simulink model "Quadruped"  (R2020a)
settings: Solver=VariableStepAuto  StartTime=0.0  StopTime=10.0  RelTol=1e-3  EnableMultiTasking=on
PreLoadFcn:
  | Parameters;
values from neighbouring files (symbols this model uses):
  buffer = 8000    [Parameters.m]
  gait_time = 1    [Parameters.m]
  l1 = 0.2    [Parameters.m]
  l2 = 0.4    [Parameters.m]
  l3 = l3_orig-r    (= 0.38)    [Parameters.m]
  robot_b = 0.1    [Parameters.m]
  robot_l = 1    [Parameters.m]
  robot_w = 0.4    [Parameters.m]
  step_height = 0.1    [Parameters.m]
  step_time = gait_time/2    (= 0.5)    [Parameters.m]
  target1 = 0    [Parameters.m]
  target2 = 30    [Parameters.m]
  target2r = -30    [Parameters.m]
  target3 = -120    [Parameters.m]
  target3r = 120    [Parameters.m]
  Xc_i = 0    [Parameters.m]
undefined symbols (not defined in the file or in its folder): X, Y, Z
libraries: sm_lib x76, nesl_utility x46, simulink x26
(part 1 of 4)
settings Model: Creator=user  LastModifiedBy=ashut
settings DataIOCC: LimitDataPoints=on  MaxDataPoints=10000
settings OptimizationCC: LifeSpan=inf
settings DebuggingCC: AllowSymbolicDim=off  SFUnexpectedBacktrackingDiag=warning  SFNoUnconditionalDefaultTransitionDiag=warning  SFExecutionAtInitializationDiag=none  ArithmeticOperatorsInVariantConditions=warning
settings SFSimCC: SimUseLocalCustomCode=off  CustomCodeUndefinedFunction=UseInterfaceOnly
settings RTWCC: RTWUseLocalCustomCode=off
settings CodeAppCC: StateflowObjectComments=on
settings GRTTargetCC: TargetLangStandard=C89/C90 (ANSI)
settings ConfigComp: CovMetricSettings=dw  CovHtmlReporting=on  CovSaveCumulativeToWorkspaceVar=on  CovSaveSingleToWorkspaceVar=on  CovExternalEMLEnable=off  CovSFcnEnable=off
settings SimscapeCC: SimscapeLogType=all  SimscapeLogSimulationStatistics=on  SimscapeLogDataHistory=10000
settings ExplorerConfigSet: InternalSimMechanicsExplorerSettings="<ExplorerConfiguration><canonicalview>default</canonicalview><AnimationSetting><BasePlaybackSpeed>1.0</BasePlaybackSpeed><PlaybackSpeedFactor>1.0</PlaybackSpeedFactor></AnimationSetting><TilePanel><TileInfo><Tiles Columns=\"1\" Count=\"1\" Rows=\"1\"><Column Weight=\"1\"/><Row Weight=\"1\"/><Tile Height=\"1\" Width=\"1\" X=\"0\" Y=\"0\"/></Tiles></TileInfo><SceneInfo><SceneViewer><BGColor><R>0.60000002384185791</R><G>0.60000002384185791</G><B>0.60000002384185791</B></BGColor><Camera><DoPerspective>off</DoPerspective><Position><X>29.2456293007888846</X><Y>-28.7629640651694523</Y><Z>29.0332714283084741</Z></Position><Center><X>0.231674806078519896</X><Y>0.250990429540917881</Y><Z>0.0193169335981059412</Z></Center><Up><X>-0.408248290463863073</X><Y>0.408248290463863073</Y><Z>0.816496580927726145</Z></Up><ViewLimDist>1</ViewLimDist><YLim>1.3149570353676332</YLim><XLim>2.00111393750615596</XLim></Camera></SceneViewer></SceneInfo></TilePanel><MechEditorPanel><Cameras/><GfxPanelCameraMap/><VideoCreator><PlaybackSpeedRatio>1.0</PlaybackSpeedRatio><FrameRate>30</FrameRate><VideoFormat>Motion JPEG AVI</VideoFormat><FrameSize>auto</FrameSize></VideoCreator></MechEditorPanel></ExplorerConfiguration>"

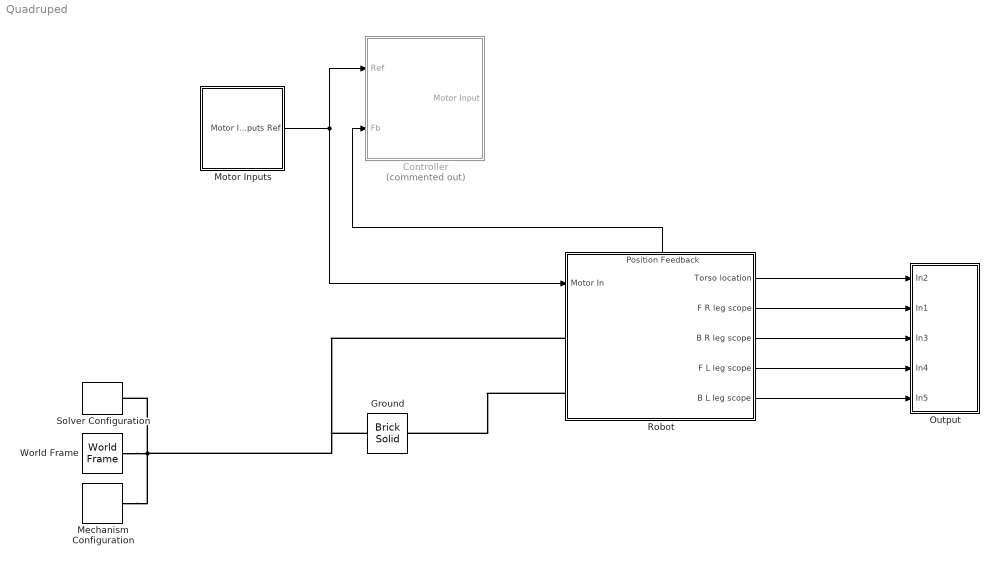
== system Quadruped ==
  Controller : Subsystem  Commented=on
  Ground : sm_lib/Body Elements/Brick Solid  GraphicAmbientColor=[0.15 0.15 0.15 1.0]  BasedOnType=Density  BrickDimensions=[100 5 0.1]  BrickDimensionUnits=m  CenterOfMass=[0 0 0]  CenterOfMassUnits=m  GraphicDiffuseColor=[0.5 0.5 0.5]  Density=1000  DensityUnits=kg/m^3  DoExposeReferenceFrame=on  GraphicEmissiveColor=[0.0 0.0 0.0 1.0]  ExportEntireGeometry=on  SerializedFrames=<Frames/>  MarkerShape=Sphere  MarkerSize=10  GraphicType=FromGeometry  InertiaType=CalculateFromGeometry  Mass=1  MassUnits=kg  MomentsOfInertia=[1 1 1]  MomentsOfInertiaUnits=kg*m^2  GraphicOpacity=1.0  ProductsOfInertia=[0 0 0]  ProductsOfInertiaUnits=kg*m^2  GraphicShininess=75  GraphicSpecularColor=[0.5 0.5 0.5 1.0]  GraphicVisPropType=SimpleVisualProperties
  Mechanism Configuration : sm_lib/Utilities/Mechanism Configuration  UniformGravity=Constant  GravityVector=[0 0 -9.8066]  GravityUnits=m/s^2  LinearizationDelta=0.001
  Motor Inputs : Subsystem
  Output : Subsystem
  Robot : Subsystem
      settings: PortSchema="{\"entries\":[{\"content\":{\"sides\":[{\"content\":{\"connectorIds\":[\"In1\",\"LConn1\",\"LConn2\"]},\"type\":\"ConnectorPlacement.EquallySpacedRectSide\",\"uuid\":\"4635b272-c60d-4014-ab6c-106026f55e73\"},{\"content\":{\"connectorIds\":[\"Out1\",\"Out2\",\"Out3\",\"Out4\",\"Out5\"],\"side\":\"RIGHT\"},\"type\":\"ConnectorPlacement.EquallySpacedRectSide\",\"uuid\":\"ef84d230-707b-4f1f-8f8a-5325fbe6d1ad\"},{\"content\":{\"connectorIds\":[\"Out6\"],\"side\":\"TOP\"},\"type\":\"ConnectorPlacement.EquallySpacedRectSide\",\"uuid\":\"c3e351c9-2d6a-4656-b5fa-3d004952b50f\"}]},\"type\":\"ConnectorPlacement.EquallySpacedConnector\",\"uuid\":\"b3bf907b-4dd7-42ee-b13b-00e04b6696fd\"}],\"packageUris\":[\"http://schema.mathworks.com/mf0/Connector/19700101\"],\"version\":\"1.0\"}"
  Solver Configuration : nesl_utility/Solver Configuration  PhysicalDomain=network_engine_domain  SubClassName=solver  LeftPortType=input  RightPortType=generic  Tones=[]  Harmonics=[]  SimulateNoise=off  Profile=off  UseLocalSampling=off  EnableSwitchedLinearOptims=on  FrequencyDomain=off  UseCCode=off  RelTol=0.001  AbsTol=1e-06  MinStep=1e-09  ToWorkspace=off  RevertToSquareIcSolve=off  NumHomotopyIterations=100  PhasorMode=off  PhasorModeNumHarmonics=1  DoDC=off  ResidualTolerance=1e-09  UseLocalSolver=off  LocalSolverChoice=NE_BACKWARD_EULER_ADVANCER  LocalSolverSampleTime=0.001  DoFixedCost=off  MaxNonlinIter=3  MaxModeIter=2  LinearAlgebra=Sparse  EquationFormulation=NE_TIME_EF  DelaysMemoryBudget=1024  AutomaticFiltering=on  FilteringTimeConstant=0.001  PartitionStorageMethod=AS_NEEDED  PartitionMemoryBudget=1024  PartitionMethod=FAST
  World Frame : sm_lib/Frames and Transforms/World Frame
  wires:
  Robot/2(F R leg scope) -> Output/2(In1)
  Robot/1(Torso location) -> Output/1(In2)
  Robot/3(B R leg scope) -> Output/3(In3)
  Robot/4(F L leg scope) -> Output/4(In4)
  Robot/5(B L leg scope) -> Output/5(In5)
  Motor Inputs/1(Motor Inputs Ref) -> Robot/1(Motor In), Controller/1(Ref)
  Robot/6(Position Feedback) -> Controller/2(Fb)
  connections:
  World Frame/RConn1 -- Ground/RConn1 -- Robot/LConn1 -- Solver Configuration/RConn1 -- Mechanism Configuration/RConn1
  Robot/LConn2 -- Ground/LConn1

== system Quadruped/Controller ==
  Ref : Inport
  Fb : Inport  Port=2
  Simple PID for each motor : Subsystem
  Motor Input : Outport
  wires:
  Ref/1 -> Simple PID for each motor/1(Ref)
  Fb/1 -> Simple PID for each motor/2(Fb)
  Simple PID for each motor/1(Motor Input) -> Motor Input/1

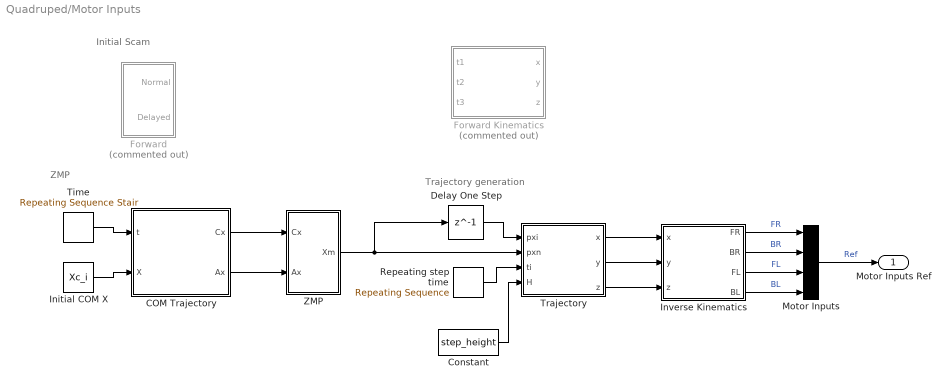
== system Quadruped/Motor Inputs ==
  note: Trajectory generation
  note: ZMP
  note: Initial Scam
  COM Trajectory : MATLAB Function  TreatAsAtomicUnit=on
  Constant : Constant  Value=step_height
  Delay One Step : Delay  DelayLength=1
  Forward : Subsystem  Commented=on
  Forward Kinematics : MATLAB Function  Commented=on  TreatAsAtomicUnit=on
  Initial COM X : Constant  Value=Xc_i
  Inverse Kinematics : Subsystem
  Motor Inputs : BusCreator  Inputs=4
  Repeating step time : simulink/Sources/Repeating Sequence  rep_seq_t=[0 step_time]  rep_seq_y=[0 step_time]
  Time : simulink/Sources/Repeating Sequence Stair  OutValues=[0:gait_time:10].'  tsamp=gait_time  OutMin=[]  OutMax=[]  OutDataTypeStr=double  OutputDataTypeScalingMode=double  OutDataType=fixdt(0,8)  ConRadixGroup=Best Precision: Vector-wise  OutScaling=2^-12
  Trajectory : MATLAB Function  TreatAsAtomicUnit=on
  ZMP : MATLAB Function  TreatAsAtomicUnit=on
  Motor Inputs Ref : Outport
  wires:
  COM Trajectory/1(Cx) -> ZMP/1(Cx)
  COM Trajectory/2(Ax) -> ZMP/2(Ax)
  Trajectory/3(z) -> Inverse Kinematics/3(z)
  Trajectory/2(y) -> Inverse Kinematics/2(y)
  Trajectory/1(x) -> Inverse Kinematics/1(x)
  Constant/1 -> Trajectory/4(H)
  Inverse Kinematics/1(FR) -> Motor Inputs/1  "FR"
  Inverse Kinematics/2(BR) -> Motor Inputs/2  "BR"
  Inverse Kinematics/3(FL) -> Motor Inputs/3  "FL"
  Inverse Kinematics/4(BL) -> Motor Inputs/4  "BL"
  Motor Inputs/1 -> Motor Inputs Ref/1  "Ref"
  Initial COM X/1 -> COM Trajectory/2(X)
  Time/1 -> COM Trajectory/1(t)
  Repeating step time/1 -> Trajectory/3(ti)
  ZMP/1(Xm) -> Delay One Step/1, Trajectory/2(pxn)
  Delay One Step/1 -> Trajectory/1(pxi)

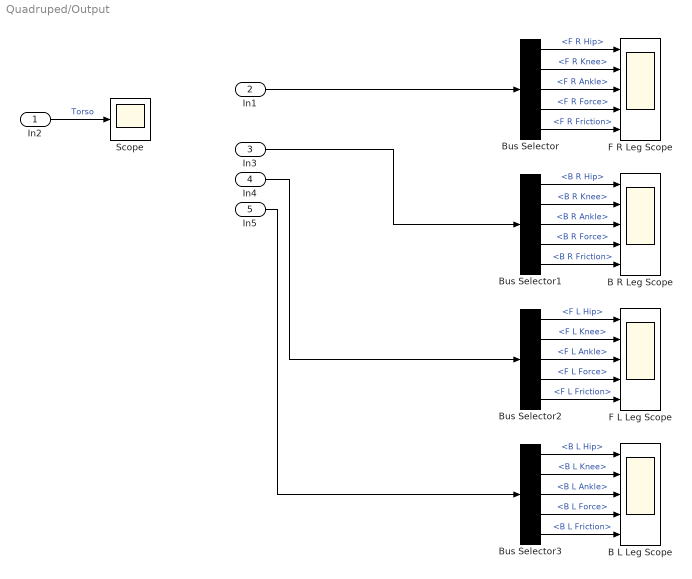
== system Quadruped/Output ==
  In2 : Inport
  In1 : Inport  Port=2
  In3 : Inport  Port=3
  In4 : Inport  Port=4
  In5 : Inport  Port=5
  B L Leg Scope : Scope  NumInputPorts=5
  B R Leg Scope : Scope  NumInputPorts=5
  Bus Selector : BusSelector  OutputSignals=Torques & Force.F R Hip,Torques & Force.F R Knee,Torques & Force.F R Ankle,Torques & Force.F R Force,Torques & Force.F R Friction
  Bus Selector1 : BusSelector  OutputSignals=Torques & Force.B R Hip,Torques & Force.B R Knee,Torques & Force.B R Ankle,Torques & Force.B R Force,Torques & Force.B R Friction
  Bus Selector2 : BusSelector  OutputSignals=Torques & Force.F L Hip,Torques & Force.F L Knee,Torques & Force.F L Ankle,Torques & Force.F L Force,Torques & Force.F L Friction
  Bus Selector3 : BusSelector  OutputSignals=Torques & Force.B L Hip,Torques & Force.B L Knee,Torques & Force.B L Ankle,Torques & Force.B L Force,Torques & Force.B L Friction
  F L Leg Scope : Scope  NumInputPorts=5
  F R Leg Scope : Scope  NumInputPorts=5
  Scope : Scope
  wires:
  Bus Selector2/2 -> F L Leg Scope/2  "<F L Knee>"
  Bus Selector3/3 -> B L Leg Scope/3  "<B L Ankle>"
  Bus Selector1/3 -> B R Leg Scope/3  "<B R Ankle>"
  Bus Selector3/2 -> B L Leg Scope/2  "<B L Knee>"
  Bus Selector1/1 -> B R Leg Scope/1  "<B R Hip>"
  In1/1 -> Bus Selector/1
  Bus Selector2/4 -> F L Leg Scope/4  "<F L Force>"
  Bus Selector1/2 -> B R Leg Scope/2  "<B R Knee>"
  Bus Selector/1 -> F R Leg Scope/1  "<F R Hip>"
  Bus Selector/3 -> F R Leg Scope/3  "<F R Ankle>"
  Bus Selector2/3 -> F L Leg Scope/3  "<F L Ankle>"
  Bus Selector/4 -> F R Leg Scope/4  "<F R Force>"
  In5/1 -> Bus Selector3/1
  Bus Selector1/4 -> B R Leg Scope/4  "<B R Force>"
  In2/1 -> Scope/1  "Torso"
  In3/1 -> Bus Selector1/1
  In4/1 -> Bus Selector2/1
  Bus Selector/2 -> F R Leg Scope/2  "<F R Knee>"
  Bus Selector3/1 -> B L Leg Scope/1  "<B L Hip>"
  Bus Selector3/4 -> B L Leg Scope/4  "<B L Force>"
  Bus Selector2/1 -> F L Leg Scope/1  "<F L Hip>"
  Bus Selector/5 -> F R Leg Scope/5  "<F R Friction>"
  Bus Selector1/5 -> B R Leg Scope/5  "<B R Friction>"
  Bus Selector2/5 -> F L Leg Scope/5  "<F L Friction>"
  Bus Selector3/5 -> B L Leg Scope/5  "<B L Friction>"

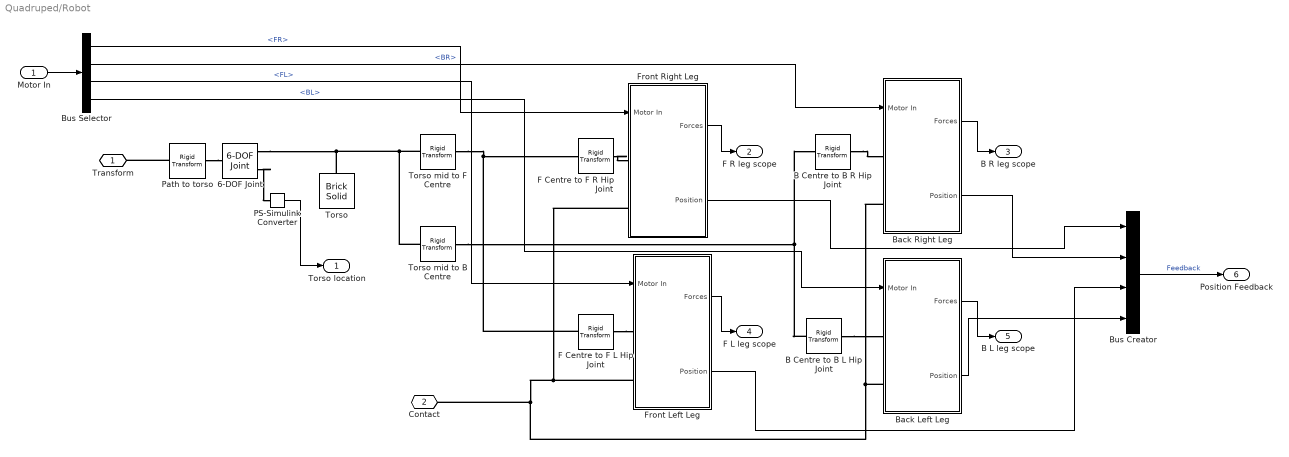
== system Quadruped/Robot ==
  Motor In : Inport
  6-DOF Joint : sm_lib/Joints/6-DOF Joint  JointMode=Normal  SenseConstraintForce=off  SenseConstraintForceX=off  SenseConstraintForceY=off  SenseConstraintForceZ=off  SenseConstraintTorque=off  SenseConstraintTorqueX=off  SenseConstraintTorqueY=off  SenseConstraintTorqueZ=off  SenseTotalForce=off  SenseTotalForceX=off  SenseTotalForceY=off  SenseTotalForceZ=off  SenseTotalTorque=off  SenseTotalTorqueX=off  SenseTotalTorqueY=off  SenseTotalTorqueZ=off  CompositeWrenchDir=FollowerOnBase  CompositeWrenchFrame=BaseFrame  PxEquilibriumPosition=0  PxEquilibriumPositionUnits=m  PxSpringStiffness=0  PxSpringStiffnessUnits=N/m  PxDampingCoefficient=0  PxDampingCoefficientUnits=N/(m/s)  PxTorqueActuationMode=NoTorque  PxMotionActuationMode=ComputedMotion  PxSensePosition=off  PxSenseVelocity=off  PxSenseAcceleration=off  PxSenseTorqueForce=off  PxSenseLowerLimitTorqueForce=off  PxSenseUpperLimitTorqueForce=off  PxLowerLimitSpecify=off  PxLowerLimitBound=-1  PxLowerLimitBoundUnits=m  PxLowerLimitStiffness=1e6  PxLowerLimitStiffnessUnits=N/m  PxLowerLimitDamping=1e3  PxLowerLimitDampingUnits=N/(m/s)  PxLowerLimitTransitionRegionWidth=1e-4  PxLowerLimitTransitionRegionWidthUnits=m  PxUpperLimitSpecify=off  PxUpperLimitBound=1  PxUpperLimitBoundUnits=m  PxUpperLimitStiffness=1e6  PxUpperLimitStiffnessUnits=N/m  PxUpperLimitDamping=1e3  PxUpperLimitDampingUnits=N/(m/s)  PxUpperLimitTransitionRegionWidth=1e-4  PxUpperLimitTransitionRegionWidthUnits=m  PxPositionTargetSpecify=off  PxPositionTargetPriority=High  PxPositionTargetValue=0  PxPositionTargetValueUnits=m  PxVelocityTargetSpecify=off  PxVelocityTargetPriority=High  PxVelocityTargetValue=0  PxVelocityTargetValueUnits=m/s  PyEquilibriumPosition=0  PyEquilibriumPositionUnits=m  PySpringStiffness=0  PySpringStiffnessUnits=N/m  PyDampingCoefficient=0  PyDampingCoefficientUnits=N/(m/s)  PyTorqueActuationMode=NoTorque  PyMotionActuationMode=ComputedMotion  PySensePosition=off  PySenseVelocity=off  PySenseAcceleration=off  PySenseTorqueForce=off  PySenseLowerLimitTorqueForce=off  PySenseUpperLimitTorqueForce=off  PyLowerLimitSpecify=off  PyLowerLimitBound=-1  PyLowerLimitBoundUnits=m  PyLowerLimitStiffness=1e6  PyLowerLimitStiffnessUnits=N/m  PyLowerLimitDamping=1e3  PyLowerLimitDampingUnits=N/(m/s)  PyLowerLimitTransitionRegionWidth=1e-4  PyLowerLimitTransitionRegionWidthUnits=m  PyUpperLimitSpecify=off  PyUpperLimitBound=1  PyUpperLimitBoundUnits=m  PyUpperLimitStiffness=1e6  PyUpperLimitStiffnessUnits=N/m  PyUpperLimitDamping=1e3  PyUpperLimitDampingUnits=N/(m/s)  PyUpperLimitTransitionRegionWidth=1e-4  PyUpperLimitTransitionRegionWidthUnits=m  PyPositionTargetSpecify=off  PyPositionTargetPriority=High  PyPositionTargetValue=0  PyPositionTargetValueUnits=m  PyVelocityTargetSpecify=off  PyVelocityTargetPriority=High  PyVelocityTargetValue=0  PyVelocityTargetValueUnits=m/s  PzEquilibriumPosition=0  PzEquilibriumPositionUnits=m  PzSpringStiffness=0  PzSpringStiffnessUnits=N/m  PzDampingCoefficient=0  PzDampingCoefficientUnits=N/(m/s)  PzTorqueActuationMode=NoTorque  PzMotionActuationMode=ComputedMotion  PzSensePosition=off  PzSenseVelocity=off  PzSenseAcceleration=off  PzSenseTorqueForce=off  PzSenseLowerLimitTorqueForce=off  PzSenseUpperLimitTorqueForce=off  PzLowerLimitSpecify=off  PzLowerLimitBound=-1  PzLowerLimitBoundUnits=m  PzLowerLimitStiffness=1e6  PzLowerLimitStiffnessUnits=N/m  PzLowerLimitDamping=1e3  PzLowerLimitDampingUnits=N/(m/s)  PzLowerLimitTransitionRegionWidth=1e-4  PzLowerLimitTransitionRegionWidthUnits=m  PzUpperLimitSpecify=off  PzUpperLimitBound=1  PzUpperLimitBoundUnits=m  PzUpperLimitStiffness=1e6  PzUpperLimitStiffnessUnits=N/m  PzUpperLimitDamping=1e3  PzUpperLimitDampingUnits=N/(m/s)  PzUpperLimitTransitionRegionWidth=1e-4  PzUpperLimitTransitionRegionWidthUnits=m  PzPositionTargetSpecify=off  PzPositionTargetPriority=High  PzPositionTargetValue=0  PzPositionTargetValueUnits=m  PzVelocityTargetSpecify=off  PzVelocityTargetPriority=High  PzVelocityTargetValue=0  PzVelocityTargetValueUnits=m/s  SphDefPosRotationMethod=None  SphDefPosRotationAngleUnits=deg  SphDefPosRotationStandardAxis=+Z  SphDefPosRotationAngle=0.0  SphDefPosRotationArbitraryAxis=[0 0 1]  SphDefPosFollAlignAxisA=+X  SphDefPosBaseAlignAxisA=+Y  SphDefPosFollAlignAxisB=+Y  SphDefPosBaseAlignAxisB=+Z  SphDefPosRotationSequenceAxes=FollowerAxes  SphDefPosRotationSequence=XYX  SphDefPosRotationSequenceAngles=[0 0 0]  SphDefPosRotationSequenceAnglesUnits=deg  SphDefPosRotationMatrix=[1 0 0; 0 1 0; 0 0 1]  SphEqPosRotationMethod=None  SphEqPosRotationAngleUnits=deg  SphEqPosRotationStandardAxis=+Z  SphEqPosRotationAngle=0.0  SphEqPosRotationArbitraryAxis=[0 0 1]  SphEqPosFollAlignAxisA=+X  SphEqPosBaseAlignAxisA=+Y  SphEqPosFollAlignAxisB=+Y  SphEqPosBaseAlignAxisB=+Z  SphEqPosRotationSequenceAxes=FollowerAxes  SphEqPosRotationSequence=XYX  SphEqPosRotationSequenceAngles=[0 0 0]  SphEqPosRotationSequenceAnglesUnits=deg  SphEqPosRotationMatrix=[1 0 0; 0 1 0; 0 0 1]  SphSpringStiffness=0  SphSpringStiffnessUnits=N*m/deg  SphDampingCoefficient=0  SphDampingCoefficientUnits=N*m/(deg/s)  SphActuateTorqueX=off  SphActuateTorqueY=off  SphActuateTorqueZ=off  SphActuateTorque=off  SphTorqueActuationMode=NoTorque  SphMotionActuationMode=ComputedMotion  SphActuationFrame=BaseFrame  SphSensePosition=on  SphSenseVelocityX=off  SphSenseVelocityY=off  SphSenseVelocityZ=off  SphSenseVelocity=off  SphSenseAccelerationX=off  SphSenseAccelerationY=off  SphSenseAccelerationZ=off  SphSenseAcceleration=off  SphSenseTorqueX=off  SphSenseTorqueY=off  SphSenseTorqueZ=off  SphSenseTorqueForce=off  SphSenseLowerLimitTorqueMag=off  SphSenseUpperLimitTorqueMag=off  SphSensingFrame=BaseFrame  SphLowerLimitSpecify=off  SphLowerLimitBound=15  SphLowerLimitBoundUnits=deg  SphLowerLimitStiffness=1e4  SphLowerLimitStiffnessUnits=N*m/deg  SphLowerLimitDamping=10  SphLowerLimitDampingUnits=N*m/(deg/s)  SphLowerLimitTransitionRegionWidth=0.1  SphLowerLimitTransitionRegionWidthUnits=deg  SphUpperLimitSpecify=off  SphUpperLimitBound=45  SphUpperLimitBoundUnits=deg  SphUpperLimitStiffness=1e4  SphUpperLimitStiffnessUnits=N*m/deg  SphUpperLimitDamping=10  SphUpperLimitDampingUnits=N*m/(deg/s)  SphUpperLimitTransitionRegionWidth=0.1  SphUpperLimitTransitionRegionWidthUnits=deg  SphPositionTargetRotationMethod=None  SphPositionTargetRotationAngleUnits=deg  SphPositionTargetRotationStandardAxis=+Z  SphPositionTargetRotationAngle=0.0  SphPositionTargetRotationArbitraryAxis=[0 0 1]  SphPositionTargetFollAlignAxisA=+X  SphPositionTargetBaseAlignAxisA=+Y  SphPositionTargetFollAlignAxisB=+Y  SphPositionTargetBaseAlignAxisB=+Z  SphPositionTargetRotationSequenceAxes=FollowerAxes  SphPositionTargetRotationSequence=XYX  SphPositionTargetRotationSequenceAngles=[0 0 0]  SphPositionTargetRotationSequenceAnglesUnits=deg  SphPositionTargetRotationMatrix=[1 0 0; 0 1 0; 0 0 1]  SphPositionTargetSpecify=off  SphPositionTargetPriority=High  SphVelocityTargetValue=[0 0 0]  SphVelocityTargetValueUnits=deg/s  SphVelocityTargetSpecify=off  SphVelocityTargetPriority=High  SphVelocityTargetInFollowerFrame=on
  B Centre to B L Hip Joint : sm_lib/Frames and Transforms/Rigid Transform  TranslationMethod=StandardAxis  TranslationStandardOffset=robot_w/2  TranslationLengthUnit=m  TranslationStandardAxis=-X  TranslationCartesianOffset=[0 0 0]  TranslationROffset=0  TranslationROffsetUnits=m  TranslationZOffset=0  TranslationZOffsetUnits=m  TranslationThetaOffset=0  TranslationThetaOffsetUnits=deg  RotationMethod=StandardAxis  RotationAngleUnits=deg  RotationStandardAxis=+Z  RotationAngle=180  RotationArbitraryAxis=[0 0 1]  FollAlignAxisA=+X  BaseAlignAxisA=+Y  FollAlignAxisB=+Y  BaseAlignAxisB=+Z  RotationSequenceAxes=FollowerAxes  RotationSequence=XYX  RotationSequenceAngles=[0 0 0]  RotationSequenceAnglesUnits=deg  RotationMatrix=[1 0 0; 0 1 0; 0 0 1]
  B Centre to B R Hip Joint : sm_lib/Frames and Transforms/Rigid Transform  TranslationMethod=StandardAxis  TranslationStandardOffset=robot_w/2  TranslationLengthUnit=m  TranslationStandardAxis=+X  TranslationCartesianOffset=[0 0 0]  TranslationROffset=0  TranslationROffsetUnits=m  TranslationZOffset=0  TranslationZOffsetUnits=m  TranslationThetaOffset=0  TranslationThetaOffsetUnits=deg  RotationMethod=None  RotationAngleUnits=deg  RotationStandardAxis=+Z  RotationAngle=0.0  RotationArbitraryAxis=[0 0 1]  FollAlignAxisA=+X  BaseAlignAxisA=+Y  FollAlignAxisB=+Y  BaseAlignAxisB=+Z  RotationSequenceAxes=FollowerAxes  RotationSequence=XYX  RotationSequenceAngles=[0 0 0]  RotationSequenceAnglesUnits=deg  RotationMatrix=[1 0 0; 0 1 0; 0 0 1]
  Back Left Leg : Subsystem
  Back Right Leg : Subsystem
  Bus Creator : BusCreator  Inputs=4
  Bus Selector : BusSelector  OutputSignals=FR,BR,FL,BL
  F Centre to F L Hip Joint : sm_lib/Frames and Transforms/Rigid Transform  TranslationMethod=StandardAxis  TranslationStandardOffset=robot_w/2  TranslationLengthUnit=m  TranslationStandardAxis=-X  TranslationCartesianOffset=[0 0 0]  TranslationROffset=0  TranslationROffsetUnits=m  TranslationZOffset=0  TranslationZOffsetUnits=m  TranslationThetaOffset=0  TranslationThetaOffsetUnits=deg  RotationMethod=StandardAxis  RotationAngleUnits=deg  RotationStandardAxis=+Z  RotationAngle=180  RotationArbitraryAxis=[0 0 1]  FollAlignAxisA=+X  BaseAlignAxisA=+Y  FollAlignAxisB=+Y  BaseAlignAxisB=+Z  RotationSequenceAxes=FollowerAxes  RotationSequence=XYX  RotationSequenceAngles=[0 0 0]  RotationSequenceAnglesUnits=deg  RotationMatrix=[1 0 0; 0 1 0; 0 0 1]
  F Centre to F R Hip Joint : sm_lib/Frames and Transforms/Rigid Transform  TranslationMethod=StandardAxis  TranslationStandardOffset=robot_w/2  TranslationLengthUnit=m  TranslationStandardAxis=+X  TranslationCartesianOffset=[0 0 0]  TranslationROffset=0  TranslationROffsetUnits=m  TranslationZOffset=0  TranslationZOffsetUnits=m  TranslationThetaOffset=0  TranslationThetaOffsetUnits=deg  RotationMethod=None  RotationAngleUnits=deg  RotationStandardAxis=+Z  RotationAngle=0.0  RotationArbitraryAxis=[0 0 1]  FollAlignAxisA=+X  BaseAlignAxisA=+Y  FollAlignAxisB=+Y  BaseAlignAxisB=+Z  RotationSequenceAxes=FollowerAxes  RotationSequence=XYX  RotationSequenceAngles=[0 0 0]  RotationSequenceAnglesUnits=deg  RotationMatrix=[1 0 0; 0 1 0; 0 0 1]
  Front Left Leg : Subsystem
  Front Right Leg : Subsystem
  PS-Simulink Converter : nesl_utility/PS-Simulink Converter  PhysicalDomain=network_engine_domain  SubClassName=ps_output  LeftPortType=input  RightPortType=output  PseudoPeriodic=off  Frequencies=[]  Unit=deg  AffineConversion=off
  Path to torso : sm_lib/Frames and Transforms/Rigid Transform  TranslationMethod=StandardAxis  TranslationStandardOffset=h  TranslationLengthUnit=m  TranslationStandardAxis=+Z  TranslationCartesianOffset=[0 0 0]  TranslationROffset=0  TranslationROffsetUnits=m  TranslationZOffset=0  TranslationZOffsetUnits=m  TranslationThetaOffset=0  TranslationThetaOffsetUnits=deg  RotationMethod=None  RotationAngleUnits=deg  RotationStandardAxis=+Z  RotationAngle=0.0  RotationArbitraryAxis=[0 0 1]  FollAlignAxisA=+X  BaseAlignAxisA=+Y  FollAlignAxisB=+Y  BaseAlignAxisB=+Z  RotationSequenceAxes=FollowerAxes  RotationSequence=XYX  RotationSequenceAngles=[0 0 0]  RotationSequenceAnglesUnits=deg  RotationMatrix=[1 0 0; 0 1 0; 0 0 1]
  Torso : sm_lib/Body Elements/Brick Solid  GraphicAmbientColor=[0.15 0.15 0.15 1.0]  BasedOnType=Density  BrickDimensions=[robot_l robot_w robot_b]  BrickDimensionUnits=m  CenterOfMass=[0 0 0]  CenterOfMassUnits=m  GraphicDiffuseColor=[0.2 0.2 1.0]  Density=density  DensityUnits=kg/m^3  DoExposeReferenceFrame=on  GraphicEmissiveColor=[0.0 0.0 0.0 1.0]  ExportEntireGeometry=off  SerializedFrames=<Frames/>  MarkerShape=Sphere  MarkerSize=10  GraphicType=FromGeometry  InertiaType=CalculateFromGeometry  Mass=1  MassUnits=kg  MomentsOfInertia=[1 1 1]  MomentsOfInertiaUnits=kg*m^2  GraphicOpacity=1.0  ProductsOfInertia=[0 0 0]  ProductsOfInertiaUnits=kg*m^2  GraphicShininess=75  GraphicSpecularColor=[0.5 0.5 0.5 1.0]  GraphicVisPropType=SimpleVisualProperties
  Torso mid to B Centre : sm_lib/Frames and Transforms/Rigid Transform  TranslationMethod=StandardAxis  TranslationStandardOffset=robot_l/2  TranslationLengthUnit=m  TranslationStandardAxis=-X  TranslationCartesianOffset=[0 0 0]  TranslationROffset=0  TranslationROffsetUnits=m  TranslationZOffset=0  TranslationZOffsetUnits=m  TranslationThetaOffset=0  TranslationThetaOffsetUnits=deg  RotationMethod=StandardAxis  RotationAngleUnits=deg  RotationStandardAxis=+Z  RotationAngle=-90.0  RotationArbitraryAxis=[0 0 1]  FollAlignAxisA=+X  BaseAlignAxisA=+Y  FollAlignAxisB=+Y  BaseAlignAxisB=+Z  RotationSequenceAxes=FollowerAxes  RotationSequence=XYX  RotationSequenceAngles=[0 0 0]  RotationSequenceAnglesUnits=deg  RotationMatrix=[1 0 0; 0 1 0; 0 0 1]
  Torso mid to F Centre : sm_lib/Frames and Transforms/Rigid Transform  TranslationMethod=StandardAxis  TranslationStandardOffset=robot_l/2  TranslationLengthUnit=m  TranslationStandardAxis=+X  TranslationCartesianOffset=[0 0 0]  TranslationROffset=0  TranslationROffsetUnits=m  TranslationZOffset=0  TranslationZOffsetUnits=m  TranslationThetaOffset=0  TranslationThetaOffsetUnits=deg  RotationMethod=StandardAxis  RotationAngleUnits=deg  RotationStandardAxis=+Z  RotationAngle=-90.0  RotationArbitraryAxis=[0 0 1]  FollAlignAxisA=+X  BaseAlignAxisA=+Y  FollAlignAxisB=+Y  BaseAlignAxisB=+Z  RotationSequenceAxes=FollowerAxes  RotationSequence=XYX  RotationSequenceAngles=[0 0 0]  RotationSequenceAnglesUnits=deg  RotationMatrix=[1 0 0; 0 1 0; 0 0 1]
  Transform : PMIOPort  Side=Left
  Contact : PMIOPort  Port=2  Side=Left
  Torso location : Outport
  F R leg scope : Outport  Port=2
  B R leg scope : Outport  Port=3
  F L leg scope : Outport  Port=4
  B L leg scope : Outport  Port=5
  Position Feedback : Outport  Port=6
  wires:
  Front Right Leg/1(Forces) -> F R leg scope/1
  PS-Simulink Converter/1 -> Torso location/1
  Back Right Leg/1(Forces) -> B R leg scope/1
  Front Left Leg/1(Forces) -> F L leg scope/1
  Back Left Leg/1(Forces) -> B L leg scope/1
  Front Right Leg/2(Position) -> Bus Creator/1
  Back Right Leg/2(Position) -> Bus Creator/2
  Front Left Leg/2(Position) -> Bus Creator/3
  Back Left Leg/2(Position) -> Bus Creator/4
  Bus Creator/1 -> Position Feedback/1  "Feedback"
  Motor In/1 -> Bus Selector/1
  Bus Selector/2 -> Back Right Leg/1(Motor In)  "<BR>"
  Bus Selector/3 -> Front Left Leg/1(Motor In)  "<FL>"
  Bus Selector/4 -> Back Left Leg/1(Motor In)  "<BL>"
  Bus Selector/1 -> Front Right Leg/1(Motor In)  "<FR>"
  connections:
  6-DOF Joint/RConn2 -- PS-Simulink Converter/LConn1
  Path to torso/RConn1 -- 6-DOF Joint/LConn1
  F Centre to F R Hip Joint/RConn1 -- Front Right Leg/LConn1
  Torso mid to F Centre/LConn1 -- Torso mid to B Centre/LConn1 -- 6-DOF Joint/RConn1 -- Torso/RConn1
  Path to torso/LConn1 -- Transform/RConn1
  Torso mid to F Centre/RConn1 -- F Centre to F L Hip Joint/LConn1 -- F Centre to F R Hip Joint/LConn1
  Front Right Leg/LConn2 -- Front Left Leg/LConn2 -- Back Right Leg/LConn2 -- Back Left Leg/LConn2 -- Contact/RConn1
  Torso mid to B Centre/RConn1 -- B Centre to B R Hip Joint/LConn1 -- B Centre to B L Hip Joint/LConn1
  B Centre to B R Hip Joint/RConn1 -- Back Right Leg/LConn1
  F Centre to F L Hip Joint/RConn1 -- Front Left Leg/LConn1
  B Centre to B L Hip Joint/RConn1 -- Back Left Leg/LConn1

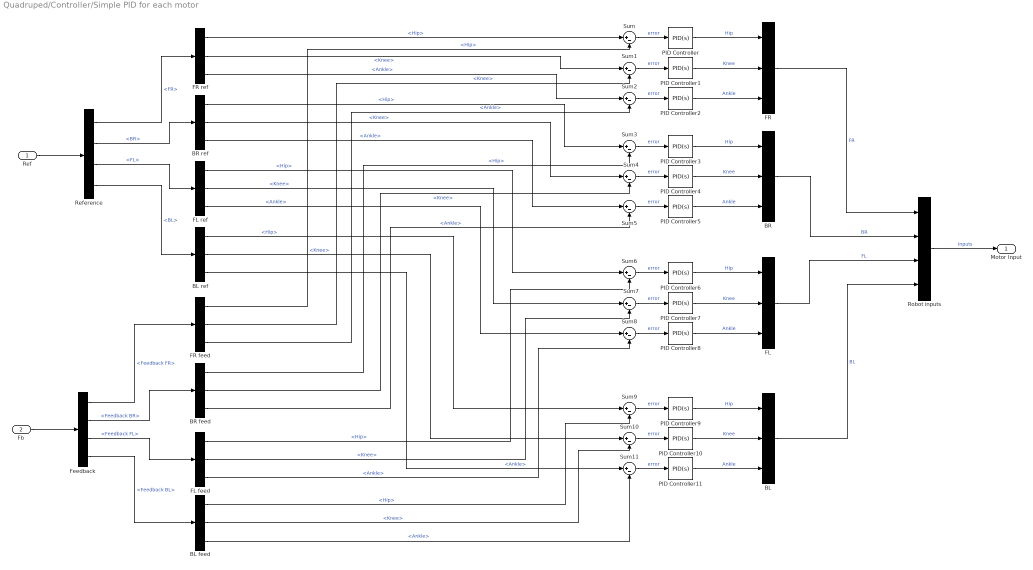
== system Quadruped/Controller/Simple PID for each motor ==
  Ref : Inport
  Fb : Inport  Port=2
  BL : BusCreator  Inputs=3
  BL feed : BusSelector  OutputSignals=Hip,Knee,Ankle
  BL ref : BusSelector  OutputSignals=Hip,Knee,Ankle
  BR : BusCreator  Inputs=3
  BR feed : BusSelector  OutputSignals=Hip,Knee,Ankle
  BR ref : BusSelector  OutputSignals=Hip,Knee,Ankle
  FL : BusCreator  Inputs=3
  FL feed : BusSelector  OutputSignals=Hip,Knee,Ankle
  FL ref : BusSelector  OutputSignals=Hip,Knee,Ankle
  FR : BusCreator  Inputs=3
  FR feed : BusSelector  OutputSignals=Hip,Knee,Ankle
  FR ref : BusSelector  OutputSignals=Hip,Knee,Ankle
  Feedback : BusSelector  OutputSignals=Feedback FR,Feedback BR,Feedback FL,Feedback BL
  PID Controller{,1..11} (12 alike) : simulink/Continuous/PID Controller  Controller=PID  Form=Parallel  TimeDomain=Continuous-time  UseExternalTs=off  SampleTime=-1  IntegratorMethod=Forward Euler  FilterMethod=Forward Euler  ControllerParametersSource=internal  P=1  I=1  D=0  UseFilter=on  N=100  TunerSelectOption=Transfer Function Based (PID Tuner App)  InitialConditionSource=internal  InitialConditionForIntegrator=0  InitialConditionForFilter=0  DifferentiatorICPrevScaledInput=0  ExternalReset=none  TrackingMode=off  Kt=1  LimitOutput=off  UpperSaturationLimit=inf  LowerSaturationLimit=-inf  LinearizeAsGain=on  AntiWindupMode=none  Kb=1  POutMin=[]  POutMax=[]  IOutMin=[]  IOutMax=[]  DOutMin=[]  DOutMax=[]  NOutMin=[]  NOutMax=[]  SumOutMin=[]  SumOutMax=[]  SaturationOutMin=[]  SaturationOutMax=[]  PParamMin=[]  PParamMax=[]  IParamMin=[]  IParamMax=[]  DParamMin=[]  DParamMax=[]  NParamMin=[]  NParamMax=[]  KbParamMin=[]  KbParamMax=[]  KtParamMin=[]  KtParamMax=[]  KbOutMin=[]  KbOutMax=[]  KtOutMin=[]  KtOutMax=[]  IntegratorOutMin=[]  IntegratorOutMax=[]  FilterOutMin=[]  FilterOutMax=[]  SumI1OutMin=[]  SumI1OutMax=[]  SumI2OutMin=[]  SumI2OutMax=[]  SumI3OutMin=[]  SumI3OutMax=[]  SumI4OutMin=[]  SumI4OutMax=[]  SumDOutMin=[]  SumDOutMax=[]  DifferentiatorOutMin=[]  DifferentiatorOutMax=[]  FilterDiffOutCoefMin=[]  FilterDiffOutCoefMax=[]  ReciprocalOutMin=[]  ReciprocalOutMax=[]  SumDenOutMin=[]  SumDenOutMax=[]  SumNumOutMin=[]  SumNumOutMax=[]  DivideOutMin=[]  DivideOutMax=[]  UdiffTsProdOutMin=[]  UdiffTsProdOutMax=[]  NTsProdOutMin=[]  NTsProdOutMax=[]  UintegralTsProdOutMin=[]  UintegralTsProdOutMax=[]  UngainTsProdOutMin=[]  UngainTsProdOutMax=[]  IntegratorContinuousStateAttributes=''  IntegratorStateMustResolveToSignalObject=off  IntegratorRTWStateStorageClass=Auto  FilterContinuousStateAttributes=''  FilterStateMustResolveToSignalObject=off  FilterRTWStateStorageClass=Auto  ParallelPVariant=InternalParameters  IdealPVariant=Disabled  IVariant=InternalParameters  DVariant=InternalParameters  IntegratorVariant=Continuous  SatVariant=Disabled  AWVariant=Passthrough  PCopyVariant=Disabled  TRVariant=Disabled  FdbkBlocksVariant=Forward  IdealPFdbkVariant=Disabled  SatFdbkVariant=Disabled  DerivativeFilterVariant=ContFilter  NVariant=InternalParameters  NCopyVariant=Disabled  FilterICVariant=InternalICsFilter  IntegratorICVariant=InternalICs  ExternalResetVariant=Disabled  TRSumVariant=Passthrough  SumFdbkVariant=Disabled  SumVariant=Sum_PID  TsampFilterVariant=InternalTs  TsampNgainVariant=Passthrough  TsampIntegralVariant=Passthrough
  Reference : BusSelector  OutputSignals=FR,BR,FL,BL
  Robot inputs : BusCreator  Inputs=4
  Sum{,1..11} (12 alike) : Sum  Inputs=|+-
  Motor Input : Outport
  wires:
  FR feed/2 -> Sum1/2  "<Knee>"
  Sum2/1 -> PID Controller2/1  "error"
  FL ref/2 -> Sum7/1  "<Knee>"
  Reference/4 -> BL ref/1  "<BL>"
  BR feed/3 -> Sum5/2  "<Ankle>"
  BL feed/3 -> Sum11/2  "<Ankle>"
  PID Controller/1 -> FR/1  "Hip"
  Feedback/4 -> BL feed/1  "<Feedback BL>"
  FL feed/3 -> Sum8/2  "<Ankle>"
  BR/1 -> Robot inputs/2  "BR"
  FR ref/2 -> Sum1/1  "<Knee>"
  Feedback/1 -> FR feed/1  "<Feedback FR>"
  Fb/1 -> Feedback/1
  FR ref/1 -> Sum/1  "<Hip>"
  PID Controller3/1 -> BR/1  "Hip"
  Sum/1 -> PID Controller/1  "error"
  FL/1 -> Robot inputs/3  "FL"
  BL/1 -> Robot inputs/4  "BL"
  Reference/3 -> FL ref/1  "<FL>"
  PID Controller7/1 -> FL/2  "Knee"
  Sum5/1 -> PID Controller5/1  "error"
  BR ref/3 -> Sum5/1  "<Ankle>"
  BL ref/3 -> Sum11/1  "<Ankle>"
  BL feed/1 -> Sum9/2  "<Hip>"
  PID Controller5/1 -> BR/3  "Ankle"
  FL feed/1 -> Sum6/2  "<Hip>"
  FR ref/3 -> Sum2/1  "<Ankle>"
  Sum7/1 -> PID Controller7/1  "error"
  Feedback/3 -> FL feed/1  "<Feedback FL>"
  Feedback/2 -> BR feed/1  "<Feedback BR>"
  Sum4/1 -> PID Controller4/1  "error"
  PID Controller10/1 -> BL/2  "Knee"
  Ref/1 -> Reference/1
  Sum11/1 -> PID Controller11/1  "error"
  BL ref/1 -> Sum9/1  "<Hip>"
  PID Controller9/1 -> BL/1  "Hip"
  PID Controller2/1 -> FR/3  "Ankle"
  FL ref/3 -> Sum8/1  "<Ankle>"
  PID Controller8/1 -> FL/3  "Ankle"
  Reference/2 -> BR ref/1  "<BR>"
  PID Controller11/1 -> BL/3  "Ankle"
  Reference/1 -> FR ref/1  "<FR>"
  Sum1/1 -> PID Controller1/1  "error"
  Sum9/1 -> PID Controller9/1  "error"
  BL feed/2 -> Sum10/2  "<Knee>"
  BL ref/2 -> Sum10/1  "<Knee>"
  FL ref/1 -> Sum6/1  "<Hip>"
  FR feed/3 -> Sum2/2  "<Ankle>"
  Sum3/1 -> PID Controller3/1  "error"
  Robot inputs/1 -> Motor Input/1  "Inputs"
  BR feed/2 -> Sum4/2  "<Knee>"
  FL feed/2 -> Sum7/2  "<Knee>"
  BR ref/2 -> Sum4/1  "<Knee>"
  PID Controller6/1 -> FL/1  "Hip"
  FR feed/1 -> Sum/2  "<Hip>"
  BR feed/1 -> Sum3/2  "<Hip>"
  Sum8/1 -> PID Controller8/1  "error"
  PID Controller4/1 -> BR/2  "Knee"
  Sum6/1 -> PID Controller6/1  "error"
  PID Controller1/1 -> FR/2  "Knee"
  Sum10/1 -> PID Controller10/1  "error"
  BR ref/1 -> Sum3/1  "<Hip>"
  FR/1 -> Robot inputs/1  "FR"

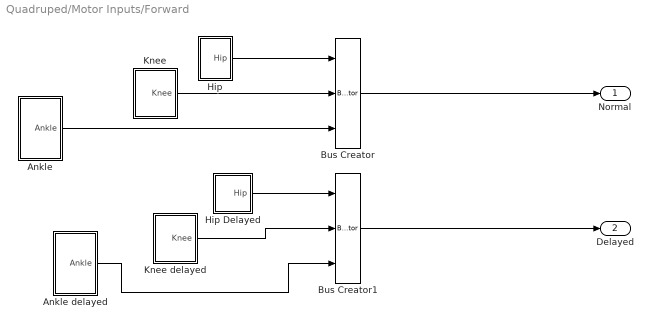
== system Quadruped/Motor Inputs/Forward ==
  Ankle : Subsystem
  Ankle delayed : Subsystem
  Bus Creator : BusCreator  Inputs=3
  Bus Creator1 : BusCreator  Inputs=3
  Hip : Subsystem
  Hip Delayed : Subsystem
  Knee : Subsystem
  Knee delayed : Subsystem
  Normal : Outport
  Delayed : Outport  Port=2
  wires:
  Knee delayed/1(Knee) -> Bus Creator1/2
  Bus Creator1/1 -> Delayed/1
  Bus Creator/1 -> Normal/1
  Hip/1(Hip) -> Bus Creator/1
  Hip Delayed/1(Hip) -> Bus Creator1/1
  Ankle delayed/1(Ankle) -> Bus Creator1/3
  Knee/1(Knee) -> Bus Creator/2
  Ankle/1(Ankle) -> Bus Creator/3

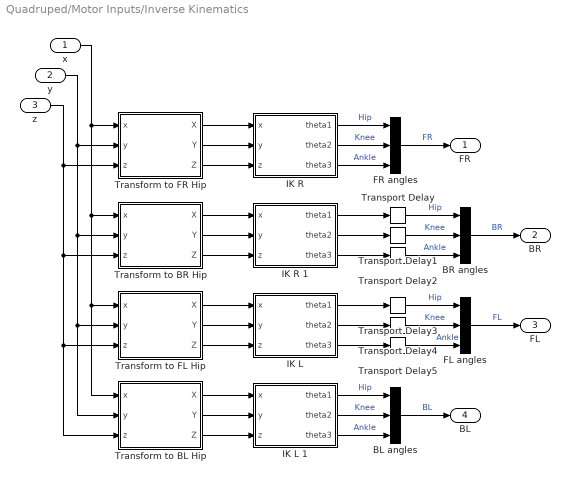
== system Quadruped/Motor Inputs/Inverse Kinematics ==
  x : Inport
  y : Inport  Port=2
  z : Inport  Port=3
  BL angles : BusCreator  Inputs=3
  BR angles : BusCreator  Inputs=3
  FL angles : BusCreator  Inputs=3
  FR angles : BusCreator  Inputs=3
  IK L : MATLAB Function  TreatAsAtomicUnit=on
  IK L 1 : MATLAB Function  TreatAsAtomicUnit=on
  IK R : MATLAB Function  TreatAsAtomicUnit=on
  IK R 1 : MATLAB Function  TreatAsAtomicUnit=on
  Transform to BL Hip : MATLAB Function  TreatAsAtomicUnit=on
  Transform to BR Hip : MATLAB Function  TreatAsAtomicUnit=on
  Transform to FL Hip : MATLAB Function  TreatAsAtomicUnit=on
  Transform to FR Hip : MATLAB Function  TreatAsAtomicUnit=on
  Transport Delay : TransportDelay  DelayTime=step_time  InitialOutput=target1
  Transport Delay1 : TransportDelay  DelayTime=step_time  InitialOutput=target2r
  Transport Delay2 : TransportDelay  DelayTime=step_time  InitialOutput=target3r
  Transport Delay3 : TransportDelay  DelayTime=step_time  InitialOutput=target1
  Transport Delay4 : TransportDelay  DelayTime=step_time  InitialOutput=target2
  Transport Delay5 : TransportDelay  DelayTime=step_time  InitialOutput=target3
  FR : Outport
  BR : Outport  Port=2
  FL : Outport  Port=3
  BL : Outport  Port=4
  wires:
  Transform to FR Hip/3(Z) -> IK R/3(z)
  Transform to FL Hip/1(X) -> IK L/1(x)
  IK L/1(theta1) -> Transport Delay3/1
  FR angles/1 -> FR/1  "FR"
  Transform to FR Hip/1(X) -> IK R/1(x)
  Transform to FR Hip/2(Y) -> IK R/2(y)
  Transform to FL Hip/2(Y) -> IK L/2(y)
  IK R/1(theta1) -> FR angles/1  "Hip"
  y/1 -> Transform to BR Hip/2(y), Transform to BL Hip/2(y), Transform to FL Hip/2(y), Transform to FR Hip/2(y)
  Transform to FL Hip/3(Z) -> IK L/3(z)
  IK L/2(theta2) -> Transport Delay4/1
  IK R/3(theta3) -> FR angles/3  "Ankle"
  IK L/3(theta3) -> Transport Delay5/1
  IK R/2(theta2) -> FR angles/2  "Knee"
  z/1 -> Transform to BR Hip/3(z), Transform to BL Hip/3(z), Transform to FL Hip/3(z), Transform to FR Hip/3(z)
  FL angles/1 -> FL/1  "FL"
  x/1 -> Transform to BR Hip/1(x), Transform to BL Hip/1(x), Transform to FL Hip/1(x), Transform to FR Hip/1(x)
  IK R 1/2(theta2) -> Transport Delay1/1
  IK R 1/3(theta3) -> Transport Delay2/1
  IK R 1/1(theta1) -> Transport Delay/1
  Transform to BR Hip/2(Y) -> IK R 1/2(y)
  Transform to BR Hip/1(X) -> IK R 1/1(x)
  BR angles/1 -> BR/1  "BR"
  Transform to BR Hip/3(Z) -> IK R 1/3(z)
  BL angles/1 -> BL/1  "BL"
  IK L 1/3(theta3) -> BL angles/3  "Ankle"
  IK L 1/2(theta2) -> BL angles/2  "Knee"
  Transform to BL Hip/3(Z) -> IK L 1/3(z)
  Transform to BL Hip/2(Y) -> IK L 1/2(y)
  IK L 1/1(theta1) -> BL angles/1  "Hip"
  Transform to BL Hip/1(X) -> IK L 1/1(x)
  Transport Delay/1 -> BR angles/1  "Hip"
  Transport Delay1/1 -> BR angles/2  "Knee"
  Transport Delay2/1 -> BR angles/3  "Ankle"
  Transport Delay3/1 -> FL angles/1  "Hip"
  Transport Delay4/1 -> FL angles/2  "Knee"
  Transport Delay5/1 -> FL angles/3  "Ankle"
